simulink model "FOSWEC_v2"  (R2022a)
settings: Solver=ode4  StartTime=0  StopTime=60  FixedStep=Ts  MaxStep=0.01  RelTol=1e-3
values from neighbouring files (symbols this model uses):
  Kt = 0.882355004501468    (= 0.882355004501)    [initModels_GUI.m]
undefined symbols (not defined in the file or in its folder): body, geometry, hydroData, pto
libraries: WECSim_Lib_PTOs x6, WECSim_Lib_Body_Elements x5, WECSim_Lib_Frames x1
settings Model: Creator=Bosma  LastModifiedBy=daquser
settings SolverCC: ConcurrentTasks=on  ZeroCrossControl=DisableAll  AlgebraicLoopSolver=TrustRegion  PositivePriorityOrder=on  AutoInsertRateTranBlk=on
settings DataIOCC: ReturnWorkspaceOutputs=off
settings OptimizationCC: BlockReduction=off  OptimizeBlockIOStorage=off  SimCompilerOptimization=on
settings DebuggingCC: TasksWithSamePriorityMsg=none  UnconnectedInputMsg=warning  UnconnectedOutputMsg=warning  UnconnectedLineMsg=warning  ModelReferenceSymbolNameMessage=none  SFMachineParentedDataDiag=warning
settings HardwareCC: ProdBitPerLong=64  ProdLongLongMode=on  ProdHWDeviceType=Intel->x86-64 (Linux 64)
settings ModelReferenceCC: ModelReferenceNumInstancesAllowed=Single
settings RTWCC: Description=Simulink Real-Time  SystemTargetFile=slrealtime.tlc  TemplateMakefile=slrealtime_default_tmf  Toolchain=Simulink Real-Time Toolchain  BuildConfiguration=Faster Runs  CodeExecutionProfiling=on  TargetLang=C++  DLArmComputeVersion=19.05
settings ExplorerConfigSet: SimMechanicsOpenEditorOnUpdate=off

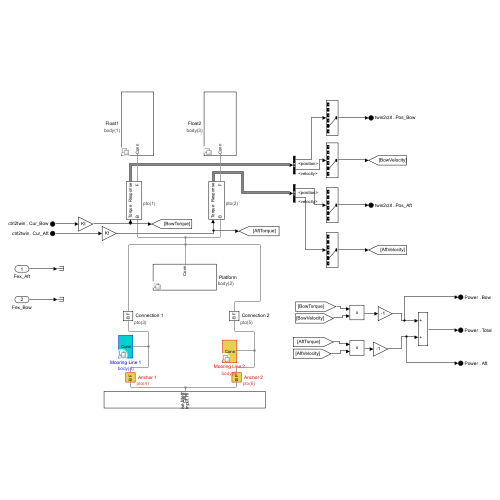
[thumbnail: Simulink's stored preview of the top-level diagram]
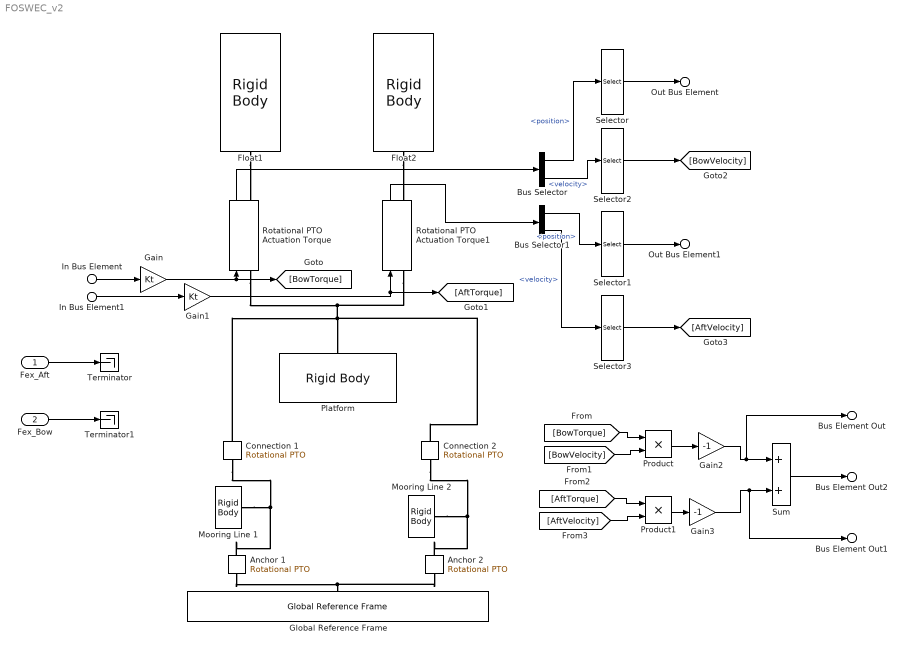
== system FOSWEC_v2 ==
  Fex_Aft : Inport
  Fex_Bow : Inport  Port=2
  In Bus Element : Inport  Port=3  PortName=ctrl2twin  Element=Cur_Bow
  In Bus Element1 : Inport  Port=3  PortName=ctrl2twin  Element=Cur_Aft
  Anchor 1 : WECSim_Lib_PTOs/Rotational PTO  pto=pto(4)  loc="0  0  0"  stiffness=0  damping=0  equilibriumPosition=0  pretension=0  displacement=0 0 0  y=0 1 0  z=0 0 1  upperLimitSpecify=off  upperLimitBound=0  upperLimitTransitionRegionWidth=0  upperLimitStiffness=0  upperLimitDamping=0  lowerLimitSpecify=off  lowerLimitBound=0  lowerLimitTransitionRegionWidth=0  lowerLimitStiffness=0  lowerLimitDamping=0
      settings: AttributesFormatString=%<pto>  SourceProductName=WEC-Sim
  Anchor 2 : WECSim_Lib_PTOs/Rotational PTO  pto=pto(6)  loc="0  0  0"  stiffness=0  damping=0  equilibriumPosition=0  pretension=0  displacement=0 0 0  y=0 1 0  z=0 0 1  upperLimitSpecify=off  upperLimitBound=0  upperLimitTransitionRegionWidth=0  upperLimitStiffness=0  upperLimitDamping=0  lowerLimitSpecify=off  lowerLimitBound=0  lowerLimitTransitionRegionWidth=0  lowerLimitStiffness=0  lowerLimitDamping=0
      settings: AttributesFormatString=%<pto>  SourceProductName=WEC-Sim
  Bus Selector : BusSelector  OutputSignals=position,velocity
  Bus Selector1 : BusSelector  OutputSignals=position,velocity
  Connection 1 : WECSim_Lib_PTOs/Rotational PTO  pto=pto(3)  loc="0  0  0"  stiffness=0  damping=0  equilibriumPosition=0  pretension=0  displacement=0 0 0  y=0 1 0  z=0 0 1  upperLimitSpecify=off  upperLimitBound=0  upperLimitTransitionRegionWidth=0  upperLimitStiffness=0  upperLimitDamping=0  lowerLimitSpecify=off  lowerLimitBound=0  lowerLimitTransitionRegionWidth=0  lowerLimitStiffness=0  lowerLimitDamping=0
      settings: AttributesFormatString=%<pto>  SourceProductName=WEC-Sim
  Connection 2 : WECSim_Lib_PTOs/Rotational PTO  pto=pto(5)  loc="0  0  0"  stiffness=0  damping=0  equilibriumPosition=0  pretension=0  displacement=0 0 0  y=0 1 0  z=0 0 1  upperLimitSpecify=off  upperLimitBound=0  upperLimitTransitionRegionWidth=0  upperLimitStiffness=0  upperLimitDamping=0  lowerLimitSpecify=off  lowerLimitBound=0  lowerLimitTransitionRegionWidth=0  lowerLimitStiffness=0  lowerLimitDamping=0
      settings: AttributesFormatString=%<pto>  SourceProductName=WEC-Sim
  Float1 : WECSim_Lib_Body_Elements/Rigid Body  body=body(1)  h5File=hydroData/*.h5  geometryFile=geometry/*.stl  mass=0  inertia=0 0 0  nonHydro=0  nonlinearHydro=0  centerGravity=0 0 0  centerBuoyancy=0 0 0  dof=6  volume=0  displacement=0 0 0  axis=0 1 0  angle=0  option=0  cd=0 0 0  ca=0 0 0  area=0 0 0  VME=0  rgME=0 0 0  z=0 0 1
  Float2 : WECSim_Lib_Body_Elements/Rigid Body  body=body(3)  h5File=hydroData/*.h5  geometryFile=geometry/*.stl  mass=0  inertia=0 0 0  nonHydro=0  nonlinearHydro=0  centerGravity=0 0 0  centerBuoyancy=0 0 0  dof=6  volume=0  displacement=0 0 0  axis=0 1 0  angle=0  option=0  cd=0 0 0  ca=0 0 0  area=0 0 0  VME=0  rgME=0 0 0  z=0 0 1
  Gain : Gain  Gain=Kt
  Gain1 : Gain  Gain=Kt
  Gain2 : Gain  Gain=-1
  Gain3 : Gain  Gain=-1
  Global Reference Frame : WECSim_Lib_Frames/Global Reference Frame  waves=waves  simu=simu  InputMethod=Input File  InputFile=wecSimInputFile.m  mode=normal  explorer=off  solver=ode4  startTime=0  rampTime=100  endTime=400  dt=0.1  cicEndTime=60  stateSpace=0  WaveClass=regular  height=2.5  period=8  elevationFile=NOT DEFINED  spectrumFile=NOT DEFINED  direction=0  spread=1  spectrumType=NOT DEFINED  phaseSeed=0  option=EqualEnergy
      settings: SourceProductName=WEC-Sim
  Mooring Line 1 : WECSim_Lib_Body_Elements/Rigid Body  body=body(4)  h5File=hydroData/*.h5  geometryFile=geometry/*.stl  mass=0  inertia=0 0 0  nonHydro=0  nonlinearHydro=0  centerGravity=0 0 0  centerBuoyancy=0 0 0  dof=6  volume=0  displacement=0 0 0  axis=0 1 0  angle=0  option=0  cd=0 0 0  ca=0 0 0  area=0 0 0  VME=0  rgME=0 0 0  z=0 0 1
      settings: SourceProductName=WEC-Sim
  Mooring Line 2 : WECSim_Lib_Body_Elements/Rigid Body  body=body(5)  h5File=hydroData/*.h5  geometryFile=geometry/*.stl  mass=0  inertia=0 0 0  nonHydro=0  nonlinearHydro=0  centerGravity=0 0 0  centerBuoyancy=0 0 0  dof=6  volume=0  displacement=0 0 0  axis=0 1 0  angle=0  option=0  cd=0 0 0  ca=0 0 0  area=0 0 0  VME=0  rgME=0 0 0  z=0 0 1
      settings: SourceProductName=WEC-Sim
  Platform : WECSim_Lib_Body_Elements/Rigid Body  body=body(2)  h5File=hydroData/*.h5  geometryFile=geometry/*.stl  mass=0  inertia=0 0 0  nonHydro=0  nonlinearHydro=0  centerGravity=0 0 0  centerBuoyancy=0 0 0  dof=6  volume=0  displacement=0 0 0  axis=0 1 0  angle=0  option=0  cd=0 0 0  ca=0 0 0  area=0 0 0  VME=0  rgME=0 0 0  z=0 0 1
  Product : Product
  Product1 : Product
  Rotational PTO Actuation Torque : WECSim_Lib_PTOs/Rotational PTO Actuation Torque  pto=pto(1)  loc="0  0  0"  stiffness=0  damping=0  equilibriumPosition=0  pretension=0  displacement=0 0 0  y=0 1 0  z=0 0 1  upperLimitSpecify=off  upperLimitBound=0  upperLimitTransitionRegionWidth=0  upperLimitStiffness=0  upperLimitDamping=0  lowerLimitSpecify=off  lowerLimitBound=0  lowerLimitTransitionRegionWidth=0  lowerLimitStiffness=0  lowerLimitDamping=0
      settings: AttributesFormatString=%<pto>  SourceProductName=WEC-Sim
  Rotational PTO Actuation Torque1 : WECSim_Lib_PTOs/Rotational PTO Actuation Torque  pto=pto(2)  loc="0  0  0"  stiffness=0  damping=0  equilibriumPosition=0  pretension=0  displacement=0 0 0  y=0 1 0  z=0 0 1  upperLimitSpecify=off  upperLimitBound=0  upperLimitTransitionRegionWidth=0  upperLimitStiffness=0  upperLimitDamping=0  lowerLimitSpecify=off  lowerLimitBound=0  lowerLimitTransitionRegionWidth=0  lowerLimitStiffness=0  lowerLimitDamping=0
      settings: AttributesFormatString=%<pto>  SourceProductName=WEC-Sim
  Selector{,1..3} (4 alike) : Selector  InputPortWidth=6  IndexOptions=Index vector (dialog)  Indices=[5]  OutputSizes=1
  Sum : Sum
  Terminator : Terminator
  Terminator1 : Terminator
  Out Bus Element : Outport  PortName=twin2ctrl  Element=Pos_Bow
  Out Bus Element1 : Outport  PortName=twin2ctrl  Element=Pos_Aft
  Bus Element Out : Outport  Port=2  PortName=Power  Element=Bow
  Bus Element Out1 : Outport  Port=2  PortName=Power  Element=Aft
  Bus Element Out2 : Outport  Port=2  PortName=Power  Element=Total
  wires:
  Rotational PTO Actuation Torque/1 -> Bus Selector/1
  Rotational PTO Actuation Torque1/1 -> Bus Selector1/1
  Bus Selector/1 -> Selector/1  "<position>"
  Bus Selector1/1 -> Selector1/1  "<position>"
  Selector/1 -> Out Bus Element/1
  Selector1/1 -> Out Bus Element1/1
  In Bus Element/1 -> Gain/1
  In Bus Element1/1 -> Gain1/1
  Fex_Aft/1 -> Terminator/1
  Fex_Bow/1 -> Terminator1/1
  Bus Selector/2 -> Selector2/1  "<velocity>"
  Bus Selector1/2 -> Selector3/1  "<velocity>"
  Gain/1 -> [BowTorque], Rotational PTO Actuation Torque/1
  Gain1/1 -> [AftTorque], Rotational PTO Actuation Torque1/1
  Selector2/1 -> [BowVelocity]
  Selector3/1 -> [AftVelocity]
  [BowVelocity] -> Product/2
  [BowTorque] -> Product/1
  [AftTorque] -> Product1/1
  [AftVelocity] -> Product1/2
  Product/1 -> Gain2/1
  Product1/1 -> Gain3/1
  Sum/1 -> Bus Element Out2/1
  Gain2/1 -> Bus Element Out/1, Sum/1
  Gain3/1 -> Bus Element Out1/1, Sum/2
  connections:
  Float1/RConn1 -- Rotational PTO Actuation Torque/RConn1
  Float2/RConn1 -- Rotational PTO Actuation Torque1/RConn1
  Connection 2/RConn1 -- Platform/RConn1 -- Connection 1/RConn1 -- Rotational PTO Actuation Torque1/LConn1 -- Rotational PTO Actuation Torque/LConn1
  Anchor 1/LConn1 -- Anchor 2/LConn1 -- Global Reference Frame/RConn1
  Connection 1/LConn1 -- Anchor 1/RConn1 -- Mooring Line 1/RConn1
  Anchor 2/RConn1 -- Connection 2/LConn1 -- Mooring Line 2/RConn1
